simulink model "MSFartoystyring27"  (R2017b)
settings: Solver=ode45  StartTime=tstart  StopTime=tstop  RelTol=1e-3  EnableMultiTasking=on
values from neighbouring files (symbols this model uses):
  c = 1    [run27.m]
  d1 = -0.0021    [init_controllers.m]
  d2 = 1.0377    [init_controllers.m]
  K = -0.0337    [init_controllers.m]
  Kd_heading = 3*lambda_heading    (= 0.3)    [init_controllers.m]
  Ki_heading = lambda_heading^3    (= 0.001)    [init_controllers.m]
  Ki_speed = lambda_speed^2    (= 0.0009)    [init_controllers.m]
  Kp_heading = 3*lambda_heading^2    (= 0.03)    [init_controllers.m]
  Kp_speed = 2*lambda_speed    (= 0.06)    [init_controllers.m]
  m = 5550    [init_controllers.m]
  omega_c = 0.1    [init_controllers.m]
  omega_n = 0.008    [init_controllers.m]
  p0 = [1500 500]    [run27.m]
  psi0 = 50*deg2rad    (= 0.872664625997)    [run27.m]
  r0 = 0    [run27.m]
  T = 62.6809    [init_controllers.m]
  target_heading_deg = atan2(WP(1,2)-WP(1,1),WP(2,2)-WP(2,1))    [run27.m]
  tsamp = 10    [run27.m]
  u_r_0 = v0(1)    [run27.m]
  U_t = 3    [run27.m]
  v0 = [6.63 0]'    [run27.m]
  zeta_c = 1    [init_controllers.m]
undefined symbols (not defined in the file or in its folder): msfartoystyring, WP
settings Model: ExtModeAutoUpdateStatusClock=off  Creator=christh  LastModifiedBy=henningward
settings SolverCC: ZeroCrossAlgorithm=Adaptive
settings DataIOCC: LimitDataPoints=on  SaveFormat=Array  SignalLoggingSaveFormat=ModelDataLogs
settings OptimizationCC: ExpressionDepthLimit=2147483647  InitFltsAndDblsToZero=on  LifeSpan=inf
settings DebuggingCC: UnderspecifiedInitializationDetection=Classic  MergeDetectMultiDrivingBlocksExec=none  MaskedZcDiagnostic=none  IgnoredZcDiagnostic=none  SolverPrmCheckMsg=warning  FcnCallInpInsideContextMsg=warning  StateNameClashWarn=warning  SFUnexpectedBacktrackingDiag=warning  SFNoUnconditionalDefaultTransitionDiag=warning  SFExecutionAtInitializationDiag=none
settings HardwareCC: ProdBitPerPointer=32  ProdBitPerSizeT=32  ProdBitPerPtrDiffT=32  ProdLargestAtomicFloat=None  ProdIntDivRoundTo=Undefined  ProdEndianess=Unspecified  ProdWordSize=32  ProdHWDeviceType=32-bit Generic
settings ModelReferenceCC: PropagateSignalLabelsOutOfModel=off
settings CodeAppCC: StateflowObjectComments=on
settings GRTTargetCC: TargetLangStandard=C89/C90 (ANSI)  GeneratePreprocessorConditionals=Disable all  CombineOutputUpdateFcns=off  GRTInterface=on
settings ConfigComp: CovMetricSettings=dw  CovHtmlReporting=on  CovSaveCumulativeToWorkspaceVar=on  CovSaveSingleToWorkspaceVar=on  CovExternalEMLEnable=off

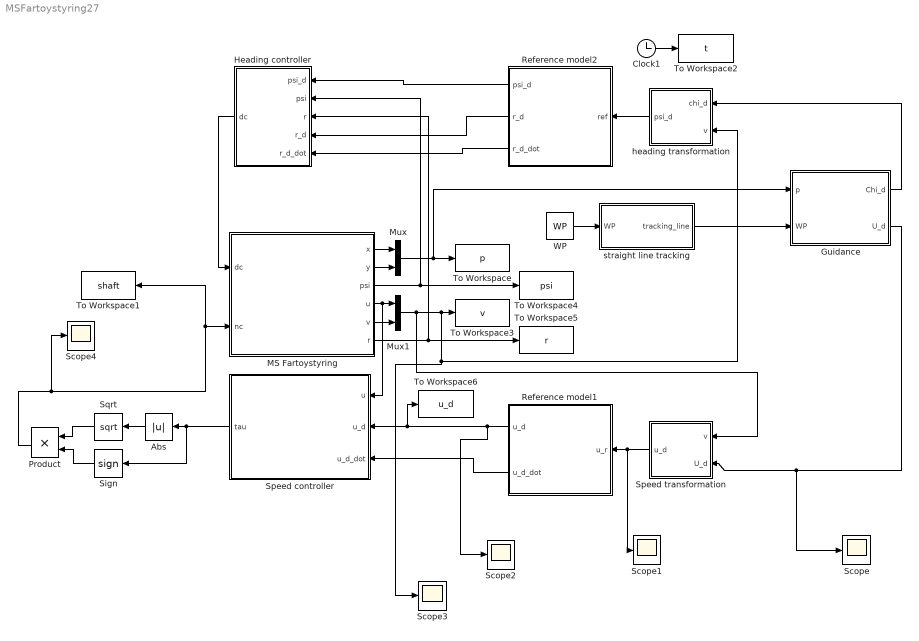
== system MSFartoystyring27 ==
  Abs : Abs
  Clock1 : Clock
  "Guidance " : Subsystem
  Heading controller : Subsystem
  MS Fartoystyring : Subsystem  mask(MS Fartoystyring for Assignment 3 G&C){x0=p0(1), y0=p0(2), u0=v0(1), v0=v0(2), psi0=psi0, r0=r0, c=c}
      mask prompts: x0 "x(t0) (m)"; y0 "y(t0) (m)"; u0 "u(t0) (m/s)"; v0 "v(t0) (m/s)"; psi0 "psi(t0) (rad)"; r0 "r(t0) (rad/s)"; c "current (0 or 1)"
      mask help:
      | Block corresponding to Figure 1 in the assignment text. Gives the response of the ship.
      |
      | The design speed of MS Fartoystyring is u=8.23 m/s.
      |
      | Input:
      | dc: commanded rudder (rad), dmax=25*pi/180
      | nc: commanded shaft speed (rad/s), nmax=85*2*pi/60
      |
      | Output:
      | x: north pos (m)
      | y: east pos (m)
      | u: surge (m/s)
      | v: sway (m/s)
      | psi: heading (rad)
      | r: yaw (rad/s)
      mask Help: Comments, bugs and help requests can be directed to the TA. Email on course website.
  Mux : Mux  Inputs=2
  Mux1 : Mux  Inputs=2
  Product : Product
  Reference model1 : Subsystem
  Reference model2 : Subsystem
  Scope{,1..4} (5 alike) : Scope
  Sign : Signum
  Speed controller : Subsystem
  Speed transformation : Subsystem
  Sqrt : Sqrt  SaturateOnIntegerOverflow=on
  To Workspace : ToWorkspace  VariableName=p  SampleTime=tsamp
  To Workspace1 : ToWorkspace  VariableName=shaft  SampleTime=tsamp
  To Workspace2 : ToWorkspace  VariableName=t  SampleTime=tsamp
  To Workspace3 : ToWorkspace  VariableName=v  SampleTime=tsamp
  To Workspace4 : ToWorkspace  VariableName=psi  SampleTime=tsamp
  To Workspace5 : ToWorkspace  VariableName=r  SampleTime=tsamp
  To Workspace6 : ToWorkspace  VariableName=u_d  SampleTime=tsamp
  WP : Constant  Value=WP
  heading transformation : Subsystem
  straight line tracking : MATLAB Function  TreatAsAtomicUnit=on
  wires:
  MS Fartoystyring/1(x) -> Mux/1
  MS Fartoystyring/2(y) -> Mux/2
  MS Fartoystyring/4(u) -> Speed controller/1("u "), Mux1/1
  MS Fartoystyring/5(v) -> Mux1/2
  Mux/1 -> "Guidance "/1(p), To Workspace/1
  Clock1/1 -> To Workspace2/1
  Speed controller/1("tau ") -> Sign/1, Abs/1
  Abs/1 -> Sqrt/1
  Sign/1 -> Product/2
  Sqrt/1 -> Product/1
  Product/1 -> Scope4/1, To Workspace1/1, MS Fartoystyring/2(nc)
  Reference model1/1(u_d) -> Scope2/1, To Workspace6/1, Speed controller/2(u_d)
  Reference model1/2(u_d_dot) -> Speed controller/3(u_d_dot)
  Reference model2/2(r_d) -> Heading controller/4(r_d)
  MS Fartoystyring/6(r) -> Heading controller/3(r), To Workspace5/1
  MS Fartoystyring/3(psi) -> Heading controller/2(psi), To Workspace4/1
  Reference model2/3("r_d_dot ") -> Heading controller/5("r_d_dot ")
  Reference model2/1(psi_d) -> Heading controller/1(psi_d)
  Heading controller/1(dc) -> MS Fartoystyring/1(dc)
  Mux1/1 -> Speed transformation/1("v "), Scope3/1, heading transformation/2(v), To Workspace3/1
  heading transformation/1("psi_d ") -> Reference model2/1(ref)
  Speed transformation/1("u_d ") -> Scope1/1, Reference model1/1(u_r)
  "Guidance "/2(U_d) -> Scope/1, Speed transformation/2("U_d ")
  WP/1 -> straight line tracking/1(WP)
  straight line tracking/1(tracking_line) -> "Guidance "/2(WP)
  "Guidance "/1("Chi_d ") -> heading transformation/1("chi_d ")

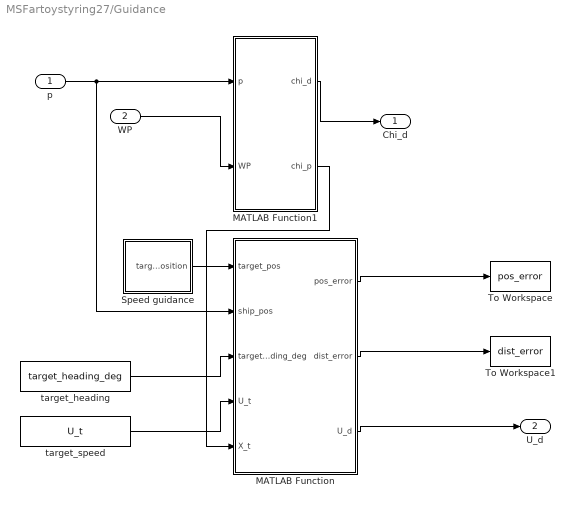
== system MSFartoystyring27/Guidance  ==
  p : Inport
  WP : Inport  Port=2
  MATLAB Function : MATLAB Function  TreatAsAtomicUnit=on
  MATLAB Function1 : MATLAB Function  TreatAsAtomicUnit=on
  Speed guidance : Subsystem
  To Workspace : ToWorkspace  VariableName=pos_error  SampleTime=tsamp
  To Workspace1 : ToWorkspace  VariableName=dist_error  SampleTime=tsamp
  target_heading : Constant  Value=target_heading_deg
  target_speed : Constant  Value=U_t
  "Chi_d " : Outport
  U_d : Outport  Port=2
  wires:
  p/1 -> MATLAB Function1/1(p), MATLAB Function/2(ship_pos)
  WP/1 -> MATLAB Function1/2(WP)
  MATLAB Function1/1(chi_d) -> "Chi_d "/1
  Speed guidance/1(target_position) -> MATLAB Function/1(target_pos)
  target_heading/1 -> MATLAB Function/3(target_heading_deg)
  MATLAB Function/3(U_d) -> U_d/1
  MATLAB Function/2(dist_error) -> To Workspace1/1
  MATLAB Function/1(pos_error) -> To Workspace/1
  target_speed/1 -> MATLAB Function/4(U_t)
  MATLAB Function1/2(chi_p) -> MATLAB Function/5(X_t)

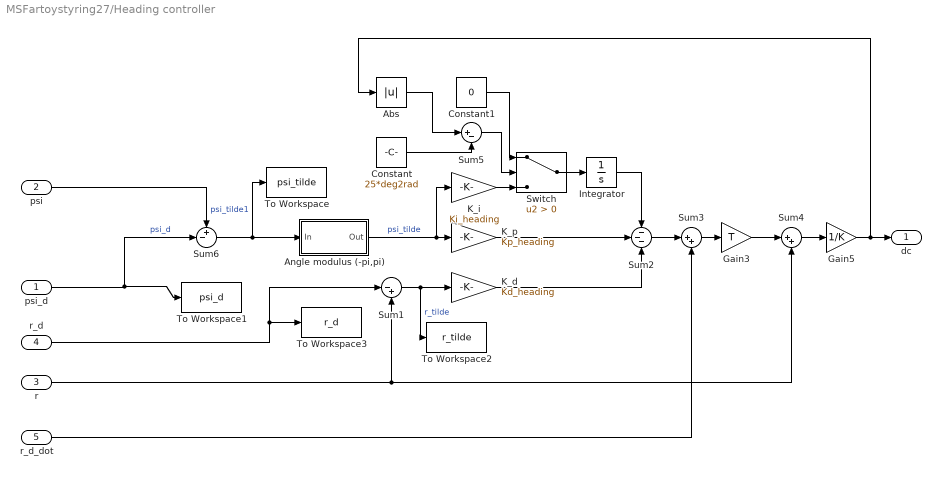
== system MSFartoystyring27/Heading controller ==
  psi_d : Inport
  psi : Inport  Port=2
  r : Inport  Port=3
  r_d : Inport  Port=4
  "r_d_dot " : Inport  Port=5
  Abs : Abs
  Angle modulus (-pi,pi) : Subsystem
  Constant : Constant  Value=25*deg2rad
  Constant1 : Constant  Value=0
  Gain3 : Gain  Gain=T
  Gain5 : Gain  Gain=1/K
  Integrator : Integrator  LimitOutput=on  UpperSaturationLimit=deg2rad*25  LowerSaturationLimit=-deg2rad*25
  K_d : Gain  Gain=Kd_heading
  K_i : Gain  Gain=Ki_heading
  K_p : Gain  Gain=Kp_heading
  Sum1 : Sum  Inputs=|-+
  Sum2 : Sum  Inputs=---
  Sum3 : Sum  Inputs=|++
  Sum4 : Sum  Inputs=|++
  Sum5 : Sum  Inputs=|+-
  Sum6 : Sum  Inputs=+-|
  Switch : Switch  Criteria=u2 > Threshold
  To Workspace : ToWorkspace  VariableName=psi_tilde  SampleTime=tsamp
  To Workspace1 : ToWorkspace  VariableName=psi_d  SampleTime=tsamp
  To Workspace2 : ToWorkspace  VariableName=r_tilde  SampleTime=tsamp
  To Workspace3 : ToWorkspace  VariableName=r_d  SampleTime=tsamp
  dc : Outport
  wires:
  Sum1/1 -> To Workspace2/1, K_d/1  "r_tilde"
  Angle modulus (-pi,pi)/1(Out) -> K_i/1, K_p/1  "psi_tilde"
  K_p/1 -> Sum2/2
  Sum2/1 -> Sum3/1
  K_d/1 -> Sum2/3
  Sum3/1 -> Gain3/1
  Gain3/1 -> Sum4/1
  r/1 -> Sum4/2, Sum1/2
  Gain5/1 -> Abs/1, dc/1
  Sum4/1 -> Gain5/1
  Integrator/1 -> Sum2/1
  Abs/1 -> Sum5/1
  Sum5/1 -> Switch/2
  Constant/1 -> Sum5/2
  Constant1/1 -> Switch/1
  K_i/1 -> Switch/3
  Switch/1 -> Integrator/1
  psi_d/1 -> To Workspace1/1, Sum6/2  "psi_d"
  Sum6/1 -> To Workspace/1, Angle modulus (-pi,pi)/1(In)  "psi_tilde1"
  psi/1 -> Sum6/1
  "r_d_dot "/1 -> Sum3/2
  r_d/1 -> To Workspace3/1, Sum1/1

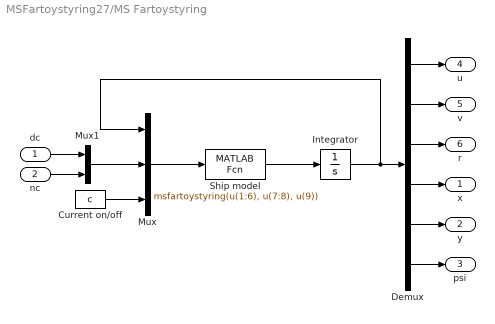
== system MSFartoystyring27/MS Fartoystyring ==
  dc : Inport
  nc : Inport  Port=2
  Current on/off : Constant  Value=c
  Demux : Demux  Outputs=6
  Integrator : Integrator  InitialCondition=[u0 v0 r0 x0 y0 psi0]'
  Mux : Mux  Inputs=3
  Mux1 : Mux  Inputs=2
  Ship model : MATLABFcn  MATLABFcn=msfartoystyring(u(1:6), u(7:8), u(9))  OutputDimensions=6
  x : Outport
  y : Outport  Port=2
  psi : Outport  Port=3
  u : Outport  Port=4
  v : Outport  Port=5
  r : Outport  Port=6
  wires:
  Integrator/1 -> Mux/1, Demux/1
  Mux1/1 -> Mux/2
  dc/1 -> Mux1/1
  nc/1 -> Mux1/2
  Demux/1 -> u/1
  Demux/2 -> v/1
  Demux/3 -> r/1
  Demux/4 -> x/1
  Demux/5 -> y/1
  Demux/6 -> psi/1
  Current on/off/1 -> Mux/3
  Ship model/1 -> Integrator/1
  Mux/1 -> Ship model/1

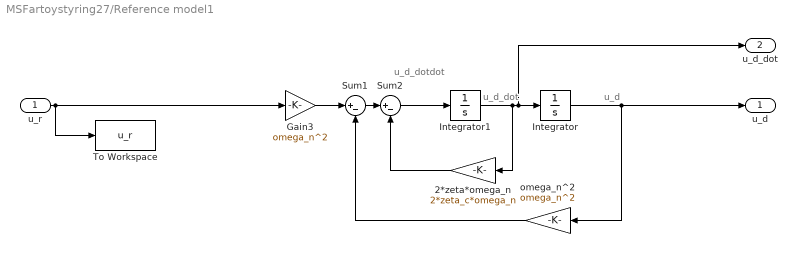
== system MSFartoystyring27/Reference model1 ==
  note: u_d
  note: u_d_dot
  note: u_d_dotdot
  u_r : Inport
  2*zeta*omega_n : Gain  Gain=2*zeta_c*omega_n
  Gain3 : Gain  Gain=omega_n^2
  Integrator : Integrator  InitialCondition=u_r_0
  Integrator1 : Integrator
  Sum1 : Sum  Inputs=|+-
  Sum2 : Sum  Inputs=|+-
  To Workspace : ToWorkspace  VariableName=u_r  SampleTime=-1
  omega_n^2 : Gain  Gain=omega_n^2
  u_d : Outport
  u_d_dot : Outport  Port=2
  wires:
  Integrator1/1 -> 2*zeta*omega_n/1, Integrator/1, u_d_dot/1
  2*zeta*omega_n/1 -> Sum2/2
  Sum1/1 -> Sum2/1
  omega_n^2/1 -> Sum1/2
  Gain3/1 -> Sum1/1
  Sum2/1 -> Integrator1/1
  Integrator/1 -> omega_n^2/1, u_d/1
  u_r/1 -> To Workspace/1, Gain3/1

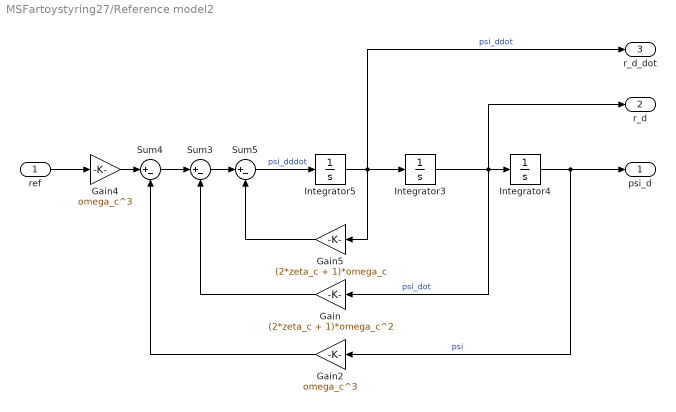
== system MSFartoystyring27/Reference model2 ==
  ref : Inport
  Gain : Gain  Gain=(2*zeta_c + 1)*omega_c^2
  Gain2 : Gain  Gain=omega_c^3
  Gain4 : Gain  Gain=omega_c^3
  Gain5 : Gain  Gain=(2*zeta_c + 1)*omega_c
  Integrator3 : Integrator
  Integrator4 : Integrator  InitialCondition=psi0
  Integrator5 : Integrator
  Sum3 : Sum  Inputs=|+-
  Sum4 : Sum  Inputs=|+-
  Sum5 : Sum  Inputs=|+-
  psi_d : Outport
  r_d : Outport  Port=2
  "r_d_dot " : Outport  Port=3
  wires:
  Integrator3/1 -> r_d/1, Gain/1, Integrator4/1  "psi_dot"
  Gain/1 -> Sum3/2
  ref/1 -> Gain4/1
  Integrator4/1 -> psi_d/1, Gain2/1  "psi"
  Sum4/1 -> Sum3/1
  Gain4/1 -> Sum4/1
  Sum3/1 -> Sum5/1
  Gain5/1 -> Sum5/2
  Sum5/1 -> Integrator5/1  "psi_dddot"
  Gain2/1 -> Sum4/2
  Integrator5/1 -> Gain5/1, "r_d_dot "/1, Integrator3/1  "psi_ddot"

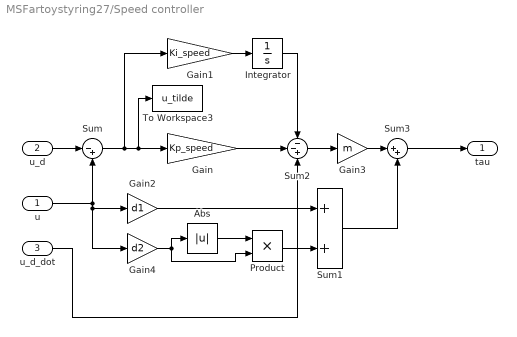
== system MSFartoystyring27/Speed controller ==
  "u " : Inport
  u_d : Inport  Port=2
  u_d_dot : Inport  Port=3
  Abs : Abs
  Gain : Gain  Gain=Kp_speed
  Gain1 : Gain  Gain=Ki_speed
  Gain2 : Gain  Gain=d1
  Gain3 : Gain  Gain=m
  Gain4 : Gain  Gain=d2
  Integrator : Integrator
  Product : Product
  Sum : Sum  Inputs=|-+
  Sum1 : Sum
  Sum2 : Sum  Inputs=--+
  Sum3 : Sum  Inputs=|++
  To Workspace3 : ToWorkspace  VariableName=u_tilde  SampleTime=tsamp
  "tau " : Outport
  wires:
  Integrator/1 -> Sum2/1
  Gain/1 -> Sum2/2
  Sum2/1 -> Gain3/1
  Gain3/1 -> Sum3/1
  u_d_dot/1 -> Sum2/3
  Sum/1 -> To Workspace3/1, Gain/1, Gain1/1
  Gain1/1 -> Integrator/1
  u_d/1 -> Sum/1
  "u "/1 -> Gain4/1, Gain2/1, Sum/2
  Abs/1 -> Product/1
  Gain4/1 -> Abs/1, Product/2
  Gain2/1 -> Sum1/1
  Product/1 -> Sum1/2
  Sum1/1 -> Sum3/2
  Sum3/1 -> "tau "/1

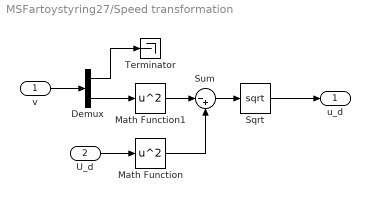
== system MSFartoystyring27/Speed transformation ==
  "v " : Inport
  "U_d " : Inport  Port=2
  Demux : Demux  Outputs=2
  Math Function : Math  Operator=square  SaturateOnIntegerOverflow=on
  Math Function1 : Math  Operator=square  SaturateOnIntegerOverflow=on
  Sqrt : Sqrt  SaturateOnIntegerOverflow=on
  Sum : Sum  Inputs=|-+
  Terminator : Terminator
  "u_d " : Outport
  wires:
  "v "/1 -> Demux/1
  Sqrt/1 -> "u_d "/1
  "U_d "/1 -> Math Function/1
  Demux/1 -> Terminator/1
  Demux/2 -> Math Function1/1
  Math Function1/1 -> Sum/1
  Math Function/1 -> Sum/2
  Sum/1 -> Sqrt/1

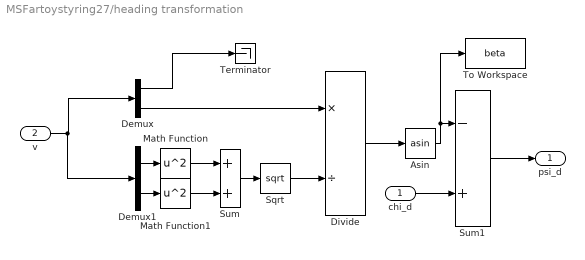
== system MSFartoystyring27/heading transformation ==
  "chi_d " : Inport
  v : Inport  Port=2
  Asin : Trigonometry  Operator=asin
  Demux : Demux  Outputs=2
  Demux1 : Demux  Outputs=2
  Divide : Product  Inputs=*/
  Math Function : Math  Operator=square  SaturateOnIntegerOverflow=on
  Math Function1 : Math  Operator=square  SaturateOnIntegerOverflow=on
  Sqrt : Sqrt  SaturateOnIntegerOverflow=on
  Sum : Sum
  Sum1 : Sum  Inputs=-+
  Terminator : Terminator
  To Workspace : ToWorkspace  VariableName=beta  SampleTime=-1
  "psi_d " : Outport
  wires:
  v/1 -> Demux1/1, Demux/1
  Demux/1 -> Terminator/1
  Demux/2 -> Divide/1
  Demux1/1 -> Math Function/1
  Demux1/2 -> Math Function1/1
  Math Function/1 -> Sum/1
  Math Function1/1 -> Sum/2
  Sum/1 -> Sqrt/1
  Sqrt/1 -> Divide/2
  Divide/1 -> Asin/1
  Asin/1 -> To Workspace/1, Sum1/1
  "chi_d "/1 -> Sum1/2
  Sum1/1 -> "psi_d "/1

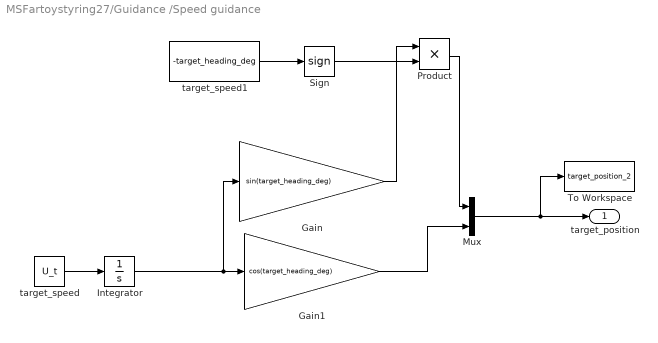
== system MSFartoystyring27/Guidance /Speed guidance ==
  Gain : Gain  Gain=sin(target_heading_deg)
  Gain1 : Gain  Gain=cos(target_heading_deg)
  Integrator : Integrator  InitialCondition=sqrt(WP(1,2)^2 + WP(2,2)^2)
  Mux : Mux  Inputs=2
  Product : Product
  Sign : Signum
  To Workspace : ToWorkspace  VariableName=target_position_2  SampleTime=tsamp
  target_speed : Constant  Value=U_t
  target_speed1 : Constant  Value=-target_heading_deg
  target_position : Outport
  wires:
  target_speed/1 -> Integrator/1
  Gain1/1 -> Mux/2
  Mux/1 -> To Workspace/1, target_position/1
  Sign/1 -> Product/2
  target_speed1/1 -> Sign/1
  Gain/1 -> Product/1
  Product/1 -> Mux/1
  Integrator/1 -> Gain1/1, Gain/1

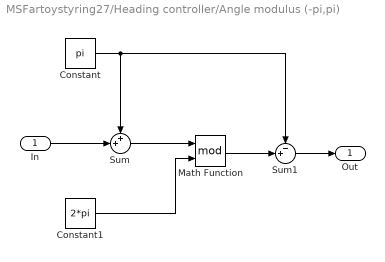
== system MSFartoystyring27/Heading controller/Angle modulus (-pi,pi) ==
  In : Inport
  Constant : Constant  Value=pi
  Constant1 : Constant  Value=2*pi
  Math Function : Math  Operator=mod  SaturateOnIntegerOverflow=on
  Sum : Sum  Inputs=++|
  Sum1 : Sum  Inputs=-+|
  Out : Outport
  wires:
  Math Function/1 -> Sum1/2
  Sum/1 -> Math Function/1
  Constant/1 -> Sum1/1, Sum/1
  In/1 -> Sum/2
  Sum1/1 -> Out/1
  Constant1/1 -> Math Function/2

== matlab function MSFartoystyring27/straight line tracking ==
  data: WP input; tracking_line output
function tracking_line = fcn(WP)
%{
tstop = 4000;
U_t = 3;
target_position = zeros(2, tstop);
target_heading_deg = [0 -1]';
target_start = WP(:,1);
target_WP = WP(:,2);
target_heading_deg(1) =-(target_WP(2)-target_start(1))/(target_WP(1)-target_start(2));
target_heading_deg = target_heading_deg / norm(target_heading_deg);
stepsize = U_t;
for i = 1:tstop/1000-1
    target_position(:, i+1) = target_position(:, i) + 1000* stepsize * target_heading_deg;
end
%}
tracking_line = WP(:,1:2);
%returning the two first waypoints for tracking.
end

== matlab function MSFartoystyring27/Guidance /MATLAB Function1 ==
  settings: updateMethod=DISCRETE  sampleTime=tsamp
  data: p input; chi_d output; WP input; chi_p output
function [chi_d,chi_p] = fcn(p, WP)
    
    %number of waypoints
    N = length(WP);
    
    % waypoint iteration
    persistent k;
    
    %waypoint iteration
    if (isempty(k))
        k = 1;
    end
    
    %reference waypoint
    xk_ref = WP(1, k);
    yk_ref = WP(2, k);
    
    %next waypoint
    xk_target = WP(1, k+1);
    yk_target = WP(2, k+1);
    
    
    if k ~= 6 && k ~= 1
        %calculating optimal turningradius
        lastWP = [WP(1,k-1); WP(2,k-1)];
        currentWP = [WP(1,k); WP(2,k)]; %way points
        nextWP = [WP(1,k+1); WP(2,k+1)];
        u = (lastWP - currentWP)/(norm(lastWP-currentWP));
        v = (nextWP - currentWP)/(norm(nextWP-currentWP)); %a,b,c
        w = (u + v)/(norm(u) + norm(v));
        a = acos((norm(v)^2 + norm(u+v)^2 - norm(u)^2)/(2*norm(v)*norm(u+v)));
        turningRadius = 900 / sin(a);
    else
        turningRadius = 900;
    end
    
   
    alpha_k = atan2(yk_target-yk_ref, xk_target-xk_ref);
    
    Rp = [cos(alpha_k) -sin(alpha_k);
          sin(alpha_k) cos(alpha_k);];
      
    epsilon = Rp'*(p - [xk_ref yk_ref]');
    
    %R = sqrt(((xk_target-xk_ref)^2+(yk_target-yk_ref)^2))-epsilon(1,:); %Radius of acceptance
    chi_p = alpha_k;
    s = epsilon(1);
    e = epsilon(2);
    
    %{
    if ((((xk_ref - p(1))^2 + (yk_ref - p(2))^2) <= 900^2) && (N > k))
        k = k + 1;
    end   
    %}
    
    Delta = 600;
    
    chi_r = atan(-e/Delta);
    chi_d = chi_p+chi_r;
    chi_d = mod(chi_d, 2*pi);
    
    
    if (norm(WP(:, k+1)-WP(:, k)) - s <= turningRadius) && (N-1 > k)
       k = k + 1;
    end
    
    
    
    
    
    
 
    
end

== matlab function MSFartoystyring27/Guidance /MATLAB Function ==
  data: target_pos input; pos_error output; ship_pos input; target_heading_deg input; dist_error output; U_t input; U_d output; X_t input
function [pos_error, dist_error, U_d]= fcn(target_pos, ship_pos, target_heading_deg, U_t, X_t)
    pos_error = ship_pos - target_pos;
    
    dist_error = sqrt(pos_error' * pos_error);
    
    R_p = [cos(target_heading_deg) -sin(target_heading_deg);
        sin(target_heading_deg) cos(target_heading_deg)];
    
    se = R_p' * pos_error;
    s = se(1) + 100; %100 = desired distance.
    e = se(2);
    max_speed = 7.26;
    Kappa = max_speed - U_t;
    Delta_s = 2000;
    
    U_d = U_t - Kappa * s/sqrt((s^2 + Delta_s^2));
    
end
